simulink model "TwinMotorGeneratorPair"  (R2021a)
settings: Solver=FixedStepAuto  StartTime=0.0  StopTime=1000  FixedStep=.01  RelTol=1e-3
undefined symbols (not defined in the file or in its folder): Ion, Li
libraries: Lib_EMTAT x12, pid_lib x3
settings Model: PacingRate=0.100000  Creator=mebell  LastModifiedBy=mebell
settings SolverCC: AlgebraicLoopSolver=TrustRegion
settings DebuggingCC: SFMachineParentedDataDiag=warning

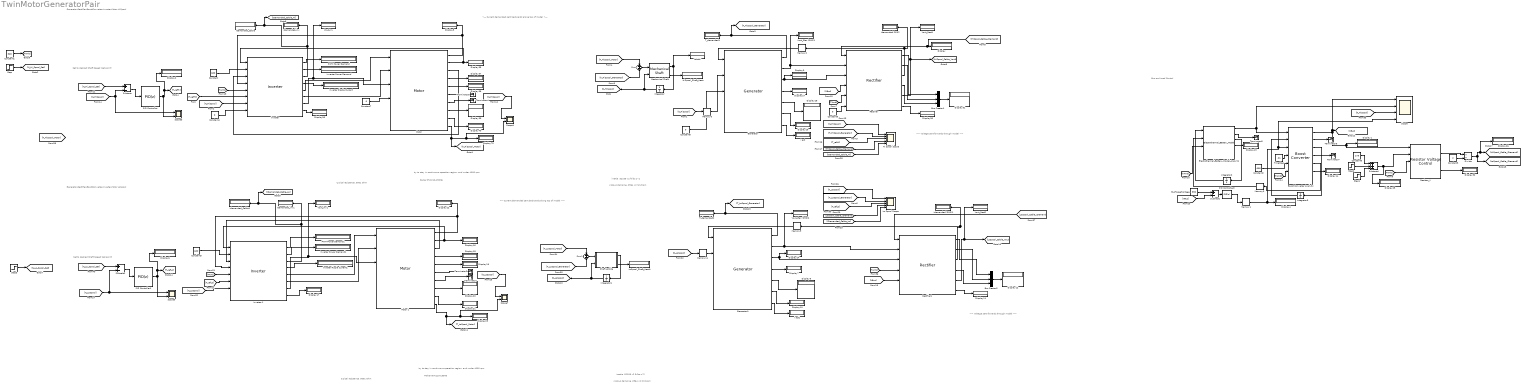
== system TwinMotorGeneratorPair ==
  note: Parker GVK210-150N6
  note: typical resistance .0001 Ohm
  note: viscous damping .2564 x2 Nm/krpm
  note: inertia .02109 x2 ft lbs s^2
  note: Set to desired Shaft Speed (set point)
  note: Generator-Rectifier-BoostConverter-Inverter-Motor HiSpool
  note: ---> Voltage sent forwards through model --->
  note: <--- Current demanded sent backwards along top of model <---
  note: try to stay in continuous operation region, and under 4000 rpm
  note: <--- Current demanded sent backwards along top of model <---
  note: Set to desired Shaft Speed (set point)
  note: Parker GVK210-150N6
  note: Generator-Rectifier-BoostConverter-Inverter-Motor LoSpool
  note: ---> Voltage sent forwards through model --->
  note: typical resistance .0001 Ohm
  note: try to stay in continuous operation region, and under 4000 rpm
  note: viscous damping .2564 x2 Nm/krpm
  note: inertia .02109 x2 ft lbs s^2
  note: Bus and Load Control
  Boost Converter Analytic : Lib_EMTAT/Components/Physics-Based/Boost Converter  Pdis_M=1  C_M=5e-08  L_M=0.00051  Ron_M=0.784  RC_M=0.26259  RL_M=0.16086  QgTotal_M=4.5e-09  Vdiode_M=0.8  TRise_M=7e-09  TFall_M=2e-09  Fsw_M=250000  Vgate_M=1.7  n_MOSFET=1  MassEst_M=0.37515  TempIn=Celsius  vOut=125  pow=100  minV=47  maxV=53  rippleMode=Use defaults (5% of voltage output and 10% of inductor current)  vRip=.05  iRip=.1  freqMode=Use default frequency (250 kHz)  freq=250e3
      link override DC - DC Converter/Steady State/TemperatureModifiedPerformanceTerm1 /Constant: Value=1
      settings: SourceProductName=EMTAT
  Bus Creator1 : BusCreator  Inputs=3
  Bus Creator2 : BusCreator  Inputs=3
  BusTargetVoltage : Constant  Value=350
  Constant : Constant  Value=600
  Constant1 : Constant  Value=528
  Constant2 : Constant  Value=.005
  Constant3 : Constant  Value=2
  Constant{4,7..9} (4 alike) : Constant  Value=0
  Constant5 : Constant  Value=600
  Constant6 : Constant  Value=175
  Display{,1..2,4..14,16..32,35..40,75} (38 alike) : Display
  Divide : Product  Inputs=*/
  Electrothermal_Battery_Model_Analytic : Lib_EMTAT/Components/Physics-Based/Electrothermal_Battery_Model  E0_M=E0_M  Q_M=Q_M  R_M=R_M  K_M=K_M  B_M=B_M  SOC_Init_M=SOC_Init_M  A_M=A_M  battery_type_M=Li-Ion  TempIn=Celsius  BWS=on  thermal=on  nameField=Thermal Model
      settings: SourceProductName=EMTAT
  Generator : Lib_EMTAT/Components/Physics-Based/Generator  pp=3  flux_m=0.38515  R_s=0.032  L_s=0.00115  P_Fe_Nom=904.3614  S_nom=4000  T_nom=70  P_out_max=22000  I_max=36.5  P_in_max=30000  T_max=80  MassEst_M=-1080970  Poles_i=6  R_s_i=.032  L_s_i=.00086+0.00029  S_nom_i=4000  T_nom_i=70  P_out_max_i=22000  I_max_i=36.5  P_in_max_i=30000  K_i=121  V_nom_i=368  T_max_i=80  CalculatePFe=Compute iron losses automatically  P_Fe_Nom_i=0  I_nom_i=36.5  PF_nom_i=0.99  P_Fe_Calc_Flag=1
      settings: SourceProductName=EMTAT
  Generator1 : Lib_EMTAT/Components/Physics-Based/Generator  pp=3  flux_m=0.38515  R_s=0.032  L_s=0.00115  P_Fe_Nom=904.3614  S_nom=4000  T_nom=70  P_out_max=22000  I_max=36.5  P_in_max=30000  T_max=80  MassEst_M=-1080970  Poles_i=6  R_s_i=.032  L_s_i=.00086+0.00029  S_nom_i=4000  T_nom_i=70  P_out_max_i=22000  I_max_i=36.5  P_in_max_i=30000  K_i=121  V_nom_i=368  T_max_i=80  CalculatePFe=Compute iron losses automatically  P_Fe_Nom_i=0  I_nom_i=36.5  PF_nom_i=0.99  P_Fe_Calc_Flag=1
      settings: SourceProductName=EMTAT
  Hi Spool Scope : Scope  NumInputPorts=5
  HiSpool_Shaft_Heat : Display
  I act : Display
  I act1 : Display
  Idemanded (RMS) : Display
  Idemanded (RMS)1 : Display
  Idemanded_Cable : Display
  Idemanded_Cable1 : Display
  Idemanded_inv : Display
  Idemanded_inv1 : Display
  Integrator : Integrator  LimitOutput=on
  Integrator1 : Integrator  LimitOutput=on
  Integrator2 : Integrator
  Integrator3 : Integrator
  "Inverter " : Lib_EMTAT/Components/Physics-Based/Inverter   T_M=[25 175]  u_D_M=[1.16666666666667 0.999999999999998]  u_ce0_M=[0.971428571428571 0.848275862068965]  R_c_M=[0.0285714285714286 0.0551724137931034]  R_D_M=[0.0238095238095238 0.0294117647058824]  E0_M=[6.00000000000002e-05 6.00000000000002e-05]  E1_M=[5.6e-05 5.6e-05]  f_sw_M=20000  L_s_M=0.1  P_max_I=22000  V_phase_I=600  f_sw_I=0  L_s_I=0.1
      settings: SourceProductName=EMTAT
  Inverter 1 : Lib_EMTAT/Components/Physics-Based/Inverter   T_M=[25 175]  u_D_M=[1.16666666666667 0.999999999999998]  u_ce0_M=[0.971428571428571 0.848275862068965]  R_c_M=[0.0285714285714286 0.0551724137931034]  R_D_M=[0.0238095238095238 0.0294117647058824]  E0_M=[6.00000000000002e-05 6.00000000000002e-05]  E1_M=[5.6e-05 5.6e-05]  f_sw_M=20000  L_s_M=0.1  P_max_I=22000  V_phase_I=600  f_sw_I=0  L_s_I=0.1
      settings: SourceProductName=EMTAT
  Inverter Power Demand : Display
  Inverter Power Demand1 : Display
  Inverter Ripple Current : Display
  Inverter Ripple Current1 : Display
  Lo Spool Scope : Scope  NumInputPorts=5
  LoSpool_Shaft_Heat1 : Display
  Mechanical Shaft : Lib_EMTAT/Components/Power Flow/Mechanical Shaft  J=0.0017575*2  B=0.0018*2
      settings: SourceProductName=EMTAT
      settings: AttributesFormatString=|
      | Mechanical Shaft
      | Version: %<LibraryVersion>
  Memory1 : Memory  InitialCondition=.8
  Memory11 : Memory  InitialCondition=3000
  Memory2 : Memory
  Memory3 : Memory  InitialCondition=.05
  Memory6 : Memory  InitialCondition=3000
  Memory9 : Memory  InitialCondition=.6
  "Motor " : Lib_EMTAT/Components/Physics-Based/Motor   pp=2.5  flux_m=0.46219  R_s=0.032  L_s=0.00115  P_Fe_Nom=904.3614  S_nom=3000  T_nom=70  P_out_max=22000  I_max=36.5  P_in_max=30000  T_max=80  MassEst_M=-1080970  Poles_i=5  R_s_i=.032  L_s_i=.00086+0.00029  S_nom_i=3000  T_nom_i=70  P_out_max_i=22000  I_max_i=36.5  P_in_max_i=30000  K_i=121  V_nom_i=368  T_max_i=80  CalculatePFe=Compute iron losses automatically  P_Fe_Nom_i=0  I_nom_i=36.5  PF_nom_i=0.99  P_Fe_Calc_Flag=1
      settings: SourceProductName=EMTAT
  Motor 1 : Lib_EMTAT/Components/Physics-Based/Motor   pp=2.5  flux_m=0.46219  R_s=0.032  L_s=0.00115  P_Fe_Nom=904.3614  S_nom=3000  T_nom=70  P_out_max=22000  I_max=36.5  P_in_max=30000  T_max=80  MassEst_M=-1080970  Poles_i=5  R_s_i=.032  L_s_i=.00086+0.00029  S_nom_i=3000  T_nom_i=70  P_out_max_i=22000  I_max_i=36.5  P_in_max_i=30000  K_i=121  V_nom_i=368  T_max_i=80  CalculatePFe=Compute iron losses automatically  P_Fe_Nom_i=0  I_nom_i=36.5  PF_nom_i=0.99  P_Fe_Calc_Flag=1
      settings: SourceProductName=EMTAT
  NdotHi : Display
  PID Controller : pid_lib/PID Controller  Controller=PID  Form=Parallel  TimeDomain=Discrete-time  UseExternalTs=off  SampleTime=-1  IntegratorMethod=Forward Euler  FilterMethod=Forward Euler  ControllerParametersSource=internal  P=0.03  I=0.008  D=0  UseFilter=off  N=48.2557908685433  TunerSelectOption=Transfer Function Based (PID Tuner App)  InitialConditionSource=internal  InitialConditionForIntegrator=0  InitialConditionForFilter=0  DifferentiatorICPrevScaledInput=0  ExternalReset=none  TrackingMode=off  Kt=1  LimitOutput=off  SatLimitsSource=internal  UpperSaturationLimit=inf  LowerSaturationLimit=-inf  LinearizeAsGain=on  AntiWindupMode=none  Kb=1  RndMeth=Round  POutMin=[]  POutMax=[]  IOutMin=[]  IOutMax=[]  DOutMin=[]  DOutMax=[]  NOutMin=[]  NOutMax=[]  SumOutMin=[]  SumOutMax=[]  SaturationOutMin=[]  SaturationOutMax=[]  PParamMin=[]  PParamMax=[]  IParamMin=[]  IParamMax=[]  DParamMin=[]  DParamMax=[]  NParamMin=[]  NParamMax=[]  KbParamMin=[]  KbParamMax=[]  KtParamMin=[]  KtParamMax=[]  KbOutMin=[]  KbOutMax=[]  KtOutMin=[]  KtOutMax=[]  IntegratorOutMin=[]  IntegratorOutMax=[]  FilterOutMin=[]  FilterOutMax=[]  SumI1OutMin=[]  SumI1OutMax=[]  SumI2OutMin=[]  SumI2OutMax=[]  SumI3OutMin=[]  SumI3OutMax=[]  SumI4OutMin=[]  SumI4OutMax=[]  SumDOutMin=[]  SumDOutMax=[]  DifferentiatorOutMin=[]  DifferentiatorOutMax=[]  FilterDiffOutCoefMin=[]  FilterDiffOutCoefMax=[]  ReciprocalOutMin=[]  ReciprocalOutMax=[]  SumDenOutMin=[]  SumDenOutMax=[]  SumNumOutMin=[]  SumNumOutMax=[]  DivideOutMin=[]  DivideOutMax=[]  UdiffTsProdOutMin=[]  UdiffTsProdOutMax=[]  NTsProdOutMin=[]  NTsProdOutMax=[]  UintegralTsProdOutMin=[]  UintegralTsProdOutMax=[]  UngainTsProdOutMin=[]  UngainTsProdOutMax=[]  IntegratorContinuousStateAttributes=''  IntegratorStateMustResolveToSignalObject=off  IntegratorRTWStateStorageClass=Auto  FilterContinuousStateAttributes=''  FilterStateMustResolveToSignalObject=off  FilterRTWStateStorageClass=Auto  ParallelPVariant=InternalParameters  IdealPVariant=Disabled  IVariant=InternalParameters  DVariant=InternalParameters  IntegratorVariant=Discrete  SatVariant=Disabled  AWVariant=Passthrough  PCopyVariant=Disabled  TRVariant=Disabled  FdbkBlocksVariant=Forward  IdealPFdbkVariant=Disabled  SatFdbkVariant=Disabled  DerivativeFilterVariant=Differentiator  NVariant=Passthrough  NCopyVariant=Disabled_SignalSpec  FilterICVariant=InternalICsDifferentiator  IntegratorICVariant=InternalICs  ExternalResetVariant=Disabled  TRSumVariant=Passthrough  SumFdbkVariant=Disabled  SumVariant=Sum_PID  TsampFilterVariant=InternalTs  TsampNgainVariant=Passthrough  TsampIntegralVariant=Passthrough  ExternalSaturationOutDataTypeStr=Inherit: Same as second input
  PID Controller1 : pid_lib/PID Controller  Controller=PID  Form=Parallel  TimeDomain=Discrete-time  UseExternalTs=off  SampleTime=-1  IntegratorMethod=Forward Euler  FilterMethod=Forward Euler  ControllerParametersSource=internal  P=0.03  I=0.008  D=0  UseFilter=off  N=48.2557908685433  TunerSelectOption=Transfer Function Based (PID Tuner App)  InitialConditionSource=internal  InitialConditionForIntegrator=0  InitialConditionForFilter=0  DifferentiatorICPrevScaledInput=0  ExternalReset=none  TrackingMode=off  Kt=1  LimitOutput=off  SatLimitsSource=internal  UpperSaturationLimit=inf  LowerSaturationLimit=-inf  LinearizeAsGain=on  AntiWindupMode=none  Kb=1  RndMeth=Round  POutMin=[]  POutMax=[]  IOutMin=[]  IOutMax=[]  DOutMin=[]  DOutMax=[]  NOutMin=[]  NOutMax=[]  SumOutMin=[]  SumOutMax=[]  SaturationOutMin=[]  SaturationOutMax=[]  PParamMin=[]  PParamMax=[]  IParamMin=[]  IParamMax=[]  DParamMin=[]  DParamMax=[]  NParamMin=[]  NParamMax=[]  KbParamMin=[]  KbParamMax=[]  KtParamMin=[]  KtParamMax=[]  KbOutMin=[]  KbOutMax=[]  KtOutMin=[]  KtOutMax=[]  IntegratorOutMin=[]  IntegratorOutMax=[]  FilterOutMin=[]  FilterOutMax=[]  SumI1OutMin=[]  SumI1OutMax=[]  SumI2OutMin=[]  SumI2OutMax=[]  SumI3OutMin=[]  SumI3OutMax=[]  SumI4OutMin=[]  SumI4OutMax=[]  SumDOutMin=[]  SumDOutMax=[]  DifferentiatorOutMin=[]  DifferentiatorOutMax=[]  FilterDiffOutCoefMin=[]  FilterDiffOutCoefMax=[]  ReciprocalOutMin=[]  ReciprocalOutMax=[]  SumDenOutMin=[]  SumDenOutMax=[]  SumNumOutMin=[]  SumNumOutMax=[]  DivideOutMin=[]  DivideOutMax=[]  UdiffTsProdOutMin=[]  UdiffTsProdOutMax=[]  NTsProdOutMin=[]  NTsProdOutMax=[]  UintegralTsProdOutMin=[]  UintegralTsProdOutMax=[]  UngainTsProdOutMin=[]  UngainTsProdOutMax=[]  IntegratorContinuousStateAttributes=''  IntegratorStateMustResolveToSignalObject=off  IntegratorRTWStateStorageClass=Auto  FilterContinuousStateAttributes=''  FilterStateMustResolveToSignalObject=off  FilterRTWStateStorageClass=Auto  ParallelPVariant=InternalParameters  IdealPVariant=Disabled  IVariant=InternalParameters  DVariant=InternalParameters  IntegratorVariant=Discrete  SatVariant=Disabled  AWVariant=Passthrough  PCopyVariant=Disabled  TRVariant=Disabled  FdbkBlocksVariant=Forward  IdealPFdbkVariant=Disabled  SatFdbkVariant=Disabled  DerivativeFilterVariant=Differentiator  NVariant=Passthrough  NCopyVariant=Disabled_SignalSpec  FilterICVariant=InternalICsDifferentiator  IntegratorICVariant=InternalICs  ExternalResetVariant=Disabled  TRSumVariant=Passthrough  SumFdbkVariant=Disabled  SumVariant=Sum_PID  TsampFilterVariant=InternalTs  TsampNgainVariant=Passthrough  TsampIntegralVariant=Passthrough  ExternalSaturationOutDataTypeStr=Inherit: Same as second input
  PID Controller2 : pid_lib/PID Controller  Controller=PID  Form=Parallel  TimeDomain=Continuous-time  UseExternalTs=off  SampleTime=-1  IntegratorMethod=Forward Euler  FilterMethod=Forward Euler  ControllerParametersSource=internal  P=.0005  I=.0003  D=0  UseFilter=on  N=0  TunerSelectOption=Transfer Function Based (PID Tuner App)  InitialConditionSource=internal  InitialConditionForIntegrator=0  InitialConditionForFilter=0  DifferentiatorICPrevScaledInput=0  ExternalReset=none  TrackingMode=off  Kt=1  LimitOutput=on  SatLimitsSource=internal  UpperSaturationLimit=1  LowerSaturationLimit=-inf  LinearizeAsGain=on  AntiWindupMode=none  Kb=1  POutMin=[]  POutMax=[]  IOutMin=[]  IOutMax=[]  DOutMin=[]  DOutMax=[]  NOutMin=[]  NOutMax=[]  SumOutMin=[]  SumOutMax=[]  SaturationOutMin=[]  SaturationOutMax=[]  PParamMin=[]  PParamMax=[]  IParamMin=[]  IParamMax=[]  DParamMin=[]  DParamMax=[]  NParamMin=[]  NParamMax=[]  KbParamMin=[]  KbParamMax=[]  KtParamMin=[]  KtParamMax=[]  KbOutMin=[]  KbOutMax=[]  KtOutMin=[]  KtOutMax=[]  IntegratorOutMin=[]  IntegratorOutMax=[]  FilterOutMin=[]  FilterOutMax=[]  SumI1OutMin=[]  SumI1OutMax=[]  SumI2OutMin=[]  SumI2OutMax=[]  SumI3OutMin=[]  SumI3OutMax=[]  SumI4OutMin=[]  SumI4OutMax=[]  SumDOutMin=[]  SumDOutMax=[]  DifferentiatorOutMin=[]  DifferentiatorOutMax=[]  FilterDiffOutCoefMin=[]  FilterDiffOutCoefMax=[]  ReciprocalOutMin=[]  ReciprocalOutMax=[]  SumDenOutMin=[]  SumDenOutMax=[]  SumNumOutMin=[]  SumNumOutMax=[]  DivideOutMin=[]  DivideOutMax=[]  UdiffTsProdOutMin=[]  UdiffTsProdOutMax=[]  NTsProdOutMin=[]  NTsProdOutMax=[]  UintegralTsProdOutMin=[]  UintegralTsProdOutMax=[]  UngainTsProdOutMin=[]  UngainTsProdOutMax=[]  IntegratorContinuousStateAttributes=''  IntegratorStateMustResolveToSignalObject=off  IntegratorRTWStateStorageClass=Auto  FilterContinuousStateAttributes=''  FilterStateMustResolveToSignalObject=off  FilterRTWStateStorageClass=Auto  ParallelPVariant=InternalParameters  IdealPVariant=Disabled  IVariant=InternalParameters  DVariant=InternalParameters  IntegratorVariant=Continuous  SatVariant=Enabled  AWVariant=Passthrough  PCopyVariant=Disabled  TRVariant=Disabled  FdbkBlocksVariant=Forward  IdealPFdbkVariant=Disabled  SatFdbkVariant=Disabled  DerivativeFilterVariant=ContFilter  NVariant=InternalParameters  NCopyVariant=Disabled  FilterICVariant=InternalICsFilter  IntegratorICVariant=InternalICs  ExternalResetVariant=Disabled  TRSumVariant=Passthrough  SumFdbkVariant=Disabled  SumVariant=Sum_PID  TsampFilterVariant=InternalTs  TsampNgainVariant=Passthrough  TsampIntegralVariant=Passthrough  ExternalSaturationOutDataTypeStr=Inherit: Same as second input
  PWM Power Demand : Display
  PWM Power Demand1 : Display
  Rectifier : Lib_EMTAT/Components/Physics-Based/Rectifier  T_M=[25 175]  u_D_M=[1.16666666666667 0.999999999999998]  u_ce0_M=[0.971428571428571 0.848275862068965]  R_c_M=[0.0285714285714286 0.0551724137931034]  R_D_M=[0.0238095238095238 0.0294117647058824]  E0_M=[6.00000000000002e-05 6.00000000000002e-05]  E1_M=[5.6e-05 5.6e-05]  f_sw_M=20000  L_s_M=0.1  P_max_I=22000  V_phase_I=600  f_sw_I=0  L_s_I=0.1
      settings: SourceProductName=EMTAT
  Rectifier1 : Lib_EMTAT/Components/Physics-Based/Rectifier  T_M=[25 175]  u_D_M=[1.16666666666667 0.999999999999998]  u_ce0_M=[0.971428571428571 0.848275862068965]  R_c_M=[0.0285714285714286 0.0551724137931034]  R_D_M=[0.0238095238095238 0.0294117647058824]  E0_M=[6.00000000000002e-05 6.00000000000002e-05]  E1_M=[5.6e-05 5.6e-05]  f_sw_M=20000  L_s_M=0.1  P_max_I=22000  V_phase_I=600  f_sw_I=0  L_s_I=0.1
      settings: SourceProductName=EMTAT
  Resistor_V : Lib_EMTAT/Components/Physics-Based/Resistor Voltage Control  TempIn=Celsius
      settings: SourceProductName=EMTAT
  Scope : Scope  NumInputPorts=4
  Scope{1,3,7,9} (4 alike) : Scope  NumInputPorts=2
  Shaft LoSide : Subsystem  mask(Mechanical Shaft){J=0.0017575*2, B=0.0018*2}
      mask prompts: J "J - Inertia, lb-ft-s^2"; B "B - Damping, lb-ft-s"
      mask help: This block models a mechanical shaft with inertia and damping effects.
      settings: AttributesFormatString=|
      | Mechanical Shaft
      | Version: %<LibraryVersion>
  Step : Step  Time=20  After=4000  SampleTime=0
  Step1 : Step  Time=120  After=172.2  SampleTime=0
  Step2 : Step  Time=500  After=1.5  SampleTime=0
  Step3 : Step  Time=10  After=4000  SampleTime=0
  Subtract : Sum  Inputs=+-
  Subtract1 : Sum  Inputs=+-
  Subtract2 : Sum  Inputs=+-
  Subtract4 : Sum  Inputs=++-
  Sum : Sum  Inputs=+|-
  Sum1 : Sum  Inputs=+|-
  T_demanded1 : Display
  T_demanded2 : Display
  Terminator{1..7} (7 alike) : Terminator
  TimeStep : Constant  Value=.01
  Vout_Gen (RMS)1 : Display
  Vout_Gen (RMS)2 : Display
  Vout_Inv : Display
  Vout_Inv1 : Display
  Vout_Rect1 : Display
  Vout_Rect2 : Display
  wires:
  "Inverter "/6 -> "Motor "/2
  Generator/4 -> Display27/1
  "Motor "/3 -> "Inverter "/3
  Constant1/1 -> [TAmb]
  "Inverter "/7 -> "Motor "/3, Vout_Inv/1
  "Motor "/2 -> "Inverter "/1, Display35/1
  "Motor "/10 -> Scope1/2, Display75/1, [T_HiSpool_Motor]  "T_HiSpool_Motor"
  "Motor "/8 -> Display39/1
  Rectifier/1 -> Bus Creator1/1
  Generator/7 -> I act/1
  [T_refHi] -> "Inverter "/6
  [TAmb] -> "Inverter "/5
  Rectifier/4 -> Bus Creator1/3
  Bus Creator1/1 -> Display31/1
  Generator/5 -> Display28/1
  Rectifier/5 -> [HiSpool_Cable_Vout], Vout_Rect1/1
  Generator/3 -> Rectifier/3, Display9/1
  [TAmb] -> Rectifier/5
  Rectifier/6 -> Display30/1
  "Motor "/5 -> Display38/1
  "Motor "/4 -> Display37/1
  "Motor "/9 -> Display40/1
  Generator/6 -> Display29/1
  Memory2/1 -> Generator/1
  [N_HiSpool] -> "Inverter "/7
  [N_HiSpool] -> Memory6/1
  "Inverter "/3 -> [IDemanded_Cable_Hi], Idemanded_Cable/1, Idemanded_inv/1
  "Inverter "/8 -> Display36/1
  Rectifier/2 -> Bus Creator1/2
  Rectifier/3 -> Idemanded (RMS)/1, Memory2/1
  "Inverter "/5 -> "Motor "/1
  Generator/1 -> [T_HiSpool_Generator], T_demanded1/1  "T_Demanded_Generator_Hi"
  Sum/1 -> Mechanical Shaft/1  "TorqueSum"
  Constant/1 -> "Inverter "/2
  [T_HiSpool_Motor] -> Sum/1
  [T_HiSpool_Generator] -> Sum/2
  Mechanical Shaft/3 -> HiSpool_Shaft_Heat/1
  [N_Hi_Spool_Set] -> Subtract/1
  [HiSpool_Cable_IDemand] -> Rectifier/1, Display/1
  "Motor "/1 -> "Inverter "/4, Display5/1
  Mechanical Shaft/1 -> Integrator/1, NdotHi/1
  Integrator/1 -> Mechanical Shaft/2, [N_HiSpool]  "N_HiSpool"
  [N_HiSpool] -> Scope1/1
  Generator/2 -> Rectifier/2, Vout_Gen (RMS)1/1
  [N_HiSpool] -> Hi Spool Scope/1  "Hi Spool Shaft Speed"
  PID Controller/1 -> Scope3/2, Display2/1, [T_refHi]
  [N_HiSpool] -> Scope3/1, Subtract/2
  Subtract/1 -> PID Controller/1
  "Inverter "/1 -> PWM Power Demand/1
  "Inverter "/2 -> Inverter Power Demand/1
  Memory6/1 -> Generator/2
  [T_refHi] -> Hi Spool Scope/3  "T_Motor Hi"
  [HiSpool_Cable_IDemand] -> Hi Spool Scope/4  "Hi Load Current Demand"
  Inverter 1/2 -> Inverter Power Demand1/1
  [N_LoSpool] -> Lo Spool Scope/1  "Lo Spool Shaft Speed"
  [LoSpool_Cable_IDemand] -> Rectifier1/1
  Rectifier1/5 -> [LoSpool_Cable_Vout], Vout_Rect2/1
  Generator1/3 -> Rectifier1/3, Display24/1
  Shaft LoSide/1(Ndot) -> Integrator1/1
  PID Controller1/1 -> Scope9/2, Display6/1, [T_refLo]
  Memory11/1 -> Generator1/2
  [TAmb] -> Rectifier1/4
  Motor 1/1 -> Inverter 1/4, Display22/1
  [LoSpool_Cable_IDemand] -> Lo Spool Scope/4  "Lo Load Current Demand"
  Generator1/2 -> Rectifier1/2, Vout_Gen (RMS)2/1
  Inverter 1/1 -> PWM Power Demand1/1
  Rectifier1/1 -> Bus Creator2/1
  [N_LoSpool] -> Subtract2/2, Scope9/1
  [N_LoSpool] -> Scope7/1
  Memory9/1 -> Generator1/1
  [T_refLo] -> Inverter 1/6
  Rectifier1/2 -> Bus Creator2/2
  Integrator1/1 -> [N_LoSpool], Shaft LoSide/2(N)  "N_HiSpool"
  [N_LoSpool] -> Inverter 1/7
  Rectifier1/4 -> Bus Creator2/3
  [T_LoSpool_Generator] -> Sum1/2
  Motor 1/10 -> Scope7/2, Display23/1, [T_LoSpool_Motor]  "T_LoSpool_Motor"
  Shaft LoSide/3(Heat) -> LoSpool_Shaft_Heat1/1
  Bus Creator2/1 -> Display12/1
  [TAmb] -> Inverter 1/5
  [T_LoSpool_Motor] -> Sum1/1
  Rectifier1/3 -> Idemanded (RMS)1/1, Memory9/1
  Motor 1/9 -> Display21/1
  Inverter 1/3 -> [IDemanded_Cable_Lo], Idemanded_Cable1/1, Idemanded_inv1/1
  [N_LoSpool] -> Memory11/1
  Inverter 1/8 -> Display17/1
  Generator1/1 -> [T_LoSpool_Generator], T_demanded2/1  "T_Demanded_Generator_Lo"
  Motor 1/5 -> Display19/1
  Inverter 1/5 -> Motor 1/1
  Motor 1/4 -> Display18/1
  Generator1/6 -> Display10/1
  Rectifier1/6 -> Display11/1
  [T_refLo] -> Lo Spool Scope/3  "T_Motor_Lo"
  Subtract2/1 -> PID Controller1/1
  Constant5/1 -> Inverter 1/2
  Motor 1/8 -> Display20/1
  Motor 1/3 -> Inverter 1/3
  Motor 1/2 -> Inverter 1/1, Display16/1
  Sum1/1 -> Shaft LoSide/1(T)  "TorqueSum"
  Inverter 1/7 -> Motor 1/3, Vout_Inv1/1
  Generator1/5 -> Display8/1
  Generator1/4 -> Display7/1
  Inverter 1/6 -> Motor 1/2
  Generator1/7 -> I act1/1
  [T_HiSpool_Generator] -> Hi Spool Scope/2  "T_Demanded_Generator_Hi"
  [T_LoSpool_Generator] -> Lo Spool Scope/2  "T_Demanded_Generator_Lo"
  Motor 1/6 -> Terminator2/1
  Motor 1/7 -> Terminator1/1
  Inverter 1/4 -> Inverter Ripple Current1/1
  "Inverter "/4 -> Inverter Ripple Current/1
  "Motor "/7 -> Terminator4/1
  "Motor "/6 -> Terminator3/1
  [TAmb] -> Electrothermal_Battery_Model_Analytic/3
  Electrothermal_Battery_Model_Analytic/1 -> Boost Converter Analytic/1, Scope/2  "Battery Voltage"
  Electrothermal_Battery_Model_Analytic/3 -> Integrator2/1
  Integrator2/1 -> Electrothermal_Battery_Model_Analytic/1
  Electrothermal_Battery_Model_Analytic/2 -> Terminator5/1
  Boost Converter Analytic/5 -> Memory3/1  "Iin"
  Boost Converter Analytic/6 -> Display14/1  "PLoss"
  Electrothermal_Battery_Model_Analytic/4 -> Display13/1
  Boost Converter Analytic/3 -> Integrator3/1
  Integrator3/1 -> Boost Converter Analytic/2
  Boost Converter Analytic/2 -> Terminator6/1
  Boost Converter Analytic/1 -> Scope/1, [VBus], Display1/1, Resistor_V/1  "VBus"
  [VBus] -> Rectifier/4
  [VBus] -> Rectifier1/5
  Subtract1/1 -> PID Controller2/1
  BusTargetVoltage/1 -> Subtract1/1
  [VBus] -> Subtract1/2
  PID Controller2/1 -> Memory1/1
  TimeStep/1 -> Boost Converter Analytic/4
  [TAmb] -> Boost Converter Analytic/6
  Boost Converter Analytic/4 -> Terminator7/1
  Constant2/1 -> Boost Converter Analytic/5
  [N_HiSpool] -> Scope/3  "ShaftSpeed"
  Constant6/1 -> Subtract4/1
  Step2/1 -> Subtract4/2
  Memory3/1 -> Electrothermal_Battery_Model_Analytic/2  "IDemand"
  Step1/1 -> Subtract4/3
  Memory1/1 -> Display4/1, Scope/4, Boost Converter Analytic/3  "DutyCycle"
  [TAmb] -> Resistor_V/3
  Resistor_V/2 -> Display32/1
  Resistor_V/1 -> Divide/1
  Constant3/1 -> Divide/2
  Divide/1 -> Display26/1, [HiSpool_Cable_IDemand], [LoSpool_Cable_IDemand]
  Subtract4/1 -> Display25/1, Resistor_V/2
  Step/1 -> [N_Hi_Spool_Set]
  [N_Lo_Spool_Set] -> Subtract2/1
  [IDemanded_Cable_Lo] -> Lo Spool Scope/5  "LoMotor_Cable_IDemanded"
  [IDemanded_Cable_Hi] -> Hi Spool Scope/5  "HiMotor_Cable_IDemanded"
  Constant4/1 -> "Inverter "/8
  Constant7/1 -> "Motor "/4
  Constant8/1 -> Generator/3
  Constant9/1 -> Rectifier/6
  Step3/1 -> [N_Lo_Spool_Set]

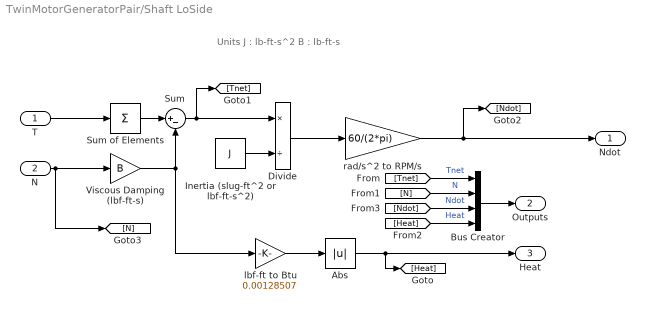
== system TwinMotorGeneratorPair/Shaft LoSide ==
  note: Units
      | J : lb-ft-s^2
      | B : lb-ft-s
  T : Inport
  N : Inport  Port=2
  Abs : Abs
  Bus Creator : BusCreator  Inputs=4
  Divide : Product  Inputs=*/
  Inertia (slug-ft^2 or lbf-ft-s^2) : Constant  Value=J
  Sum : Sum  Inputs=|+-
  Sum of Elements : Sum  Inputs=+
  Viscous Damping (lbf-ft-s) : Gain  Gain=B
  lbf-ft to Btu : Gain  Gain=0.00128507
  rad/s^2 to RPM/s : Gain  Gain=60/(2*pi)
  Ndot : Outport
  Outputs : Outport  Port=2
  Heat : Outport  Port=3
  wires:
  lbf-ft to Btu/1 -> Abs/1
  Viscous Damping (lbf-ft-s)/1 -> Sum/2, lbf-ft to Btu/1
  Sum/1 -> Divide/1, [Tnet]
  Abs/1 -> [Heat], Heat/1
  [Heat] -> Bus Creator/4  "Heat"
  [N] -> Bus Creator/2  "N"
  [Tnet] -> Bus Creator/1  "Tnet"
  T/1 -> Sum of Elements/1
  Divide/1 -> rad/s^2 to RPM/s/1
  Sum of Elements/1 -> Sum/1
  rad/s^2 to RPM/s/1 -> [Ndot], Ndot/1
  Bus Creator/1 -> Outputs/1
  Inertia (slug-ft^2 or lbf-ft-s^2)/1 -> Divide/2
  N/1 -> [N], Viscous Damping (lbf-ft-s)/1
  [Ndot] -> Bus Creator/3  "Ndot"
